simulink model "Inverse_Forward_Simscape"  (R2024b)
settings: Solver=VariableStepAuto  StartTime=0.0  StopTime=10.0  RelTol=1e-3
undefined symbols (not defined in the file or in its folder): smiData, X, Y, Z
libraries: sm_lib x70, nesl_utility x38, robotcorelib x3
(part 2 of 2)

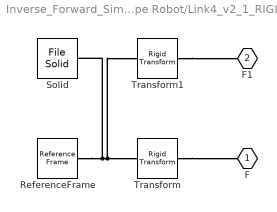
== system Inverse_Forward_Simscape/Simscape Robot/Link4_v2_1_RIGID1 ==
  ReferenceFrame : sm_lib/Frames and Transforms/Reference Frame
  Solid : sm_lib/Body Elements/File Solid  ExtGeomFileName=C:\Users\Chhay\Desktop\simscape\simscape\Solidworks FIle\Link4_v2_Default_sldprt.STEP  UnitType=FromFile  ExtGeomFileUnits=m  StepReaderType=HEX  ExportConvexHullGeometry=off  InertiaType=Custom  BasedOnType=DensityFromFile  Density=1000  DensityUnits=kg/m^3  Mass=smiData.Solid(7).mass  MassUnits=kg  CenterOfMass=smiData.Solid(7).CoM  CenterOfMassUnits=mm  MomentsOfInertia=smiData.Solid(7).MoI  MomentsOfInertiaUnits=kg*mm^2  ProductsOfInertia=smiData.Solid(7).PoI  ProductsOfInertiaUnits=kg*mm^2  GraphicType=FromGeometry  MarkerShape=Sphere  MarkerSize=10  GraphicVisPropType=SimpleVisualProperties  GraphicDiffuseColor=[0.0 1.0 1.0]  GraphicOpacity=smiData.Solid(7).opacity  GraphicSpecularColor=[0.1 0.1 0.1 1.0]  GraphicAmbientColor=[0.15 0.15 0.15 1.0]  GraphicEmissiveColor=[0.5 0.5 0.5 1.0]  GraphicShininess=75  DoExposeReferenceFrame=on  SerializedFrames=<Frames/>
  Transform : sm_lib/Frames and Transforms/Rigid Transform  RotationMethod=ArbitraryAxis  FollAlignAxisA=+X  BaseAlignAxisA=+Y  FollAlignAxisB=+Y  BaseAlignAxisB=+Z  RotationStandardAxis=+Z  RotationAngle=smiData.RigidTransform(2).angle  RotationAngleUnits=rad  RotationArbitraryAxis=smiData.RigidTransform(2).axis  RotationSequenceAxes=FollowerAxes  RotationSequence=XYX  RotationSequenceAngles=[0 0 0]  RotationSequenceAnglesUnits=deg  RotationMatrix=[1 0 0; 0 1 0; 0 0 1]  Quaternion=[1 0 0 0]  TranslationMethod=Cartesian  TranslationCartesianOffset=smiData.RigidTransform(2).translation  TranslationCartesianOffsetUnits=mm  TranslationStandardAxis=+Z  TranslationStandardOffset=0  TranslationStandardOffsetUnits=mm  TranslationROffset=0  TranslationROffsetUnits=m  TranslationThetaOffset=0  TranslationThetaOffsetUnits=deg  TranslationZOffset=0  TranslationZOffsetUnits=m
  Transform1 : sm_lib/Frames and Transforms/Rigid Transform  RotationMethod=ArbitraryAxis  FollAlignAxisA=+X  BaseAlignAxisA=+Y  FollAlignAxisB=+Y  BaseAlignAxisB=+Z  RotationStandardAxis=+Z  RotationAngle=smiData.RigidTransform(3).angle  RotationAngleUnits=rad  RotationArbitraryAxis=smiData.RigidTransform(3).axis  RotationSequenceAxes=FollowerAxes  RotationSequence=XYX  RotationSequenceAngles=[0 0 0]  RotationSequenceAnglesUnits=deg  RotationMatrix=[1 0 0; 0 1 0; 0 0 1]  Quaternion=[1 0 0 0]  TranslationMethod=Cartesian  TranslationCartesianOffset=smiData.RigidTransform(3).translation  TranslationCartesianOffsetUnits=mm  TranslationStandardAxis=+Z  TranslationStandardOffset=0  TranslationStandardOffsetUnits=mm  TranslationROffset=0  TranslationROffsetUnits=m  TranslationThetaOffset=0  TranslationThetaOffsetUnits=deg  TranslationZOffset=0  TranslationZOffsetUnits=m
  F : PMIOPort  Side=Left
  F1 : PMIOPort  Port=2  Side=Right
  connections:
  ReferenceFrame/RConn1 -- Transform/LConn1 -- Transform1/LConn1 -- Solid/RConn1
  Transform/RConn1 -- F/RConn1
  Transform1/RConn1 -- F1/RConn1

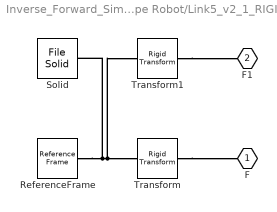
== system Inverse_Forward_Simscape/Simscape Robot/Link5_v2_1_RIGID1 ==
  ReferenceFrame : sm_lib/Frames and Transforms/Reference Frame
  Solid : sm_lib/Body Elements/File Solid  ExtGeomFileName=C:\Users\Chhay\Desktop\simscape\simscape\Solidworks FIle\Link5_v2_Default_sldprt.STEP  UnitType=FromFile  ExtGeomFileUnits=m  StepReaderType=HEX  ExportConvexHullGeometry=off  InertiaType=Custom  BasedOnType=DensityFromFile  Density=1000  DensityUnits=kg/m^3  Mass=smiData.Solid(1).mass  MassUnits=kg  CenterOfMass=smiData.Solid(1).CoM  CenterOfMassUnits=mm  MomentsOfInertia=smiData.Solid(1).MoI  MomentsOfInertiaUnits=kg*mm^2  ProductsOfInertia=smiData.Solid(1).PoI  ProductsOfInertiaUnits=kg*mm^2  GraphicType=FromGeometry  MarkerShape=Sphere  MarkerSize=10  GraphicVisPropType=SimpleVisualProperties  GraphicDiffuseColor=[0.2 1.0 1.0]  GraphicOpacity=smiData.Solid(1).opacity  GraphicSpecularColor=[0.5 0.5 0.5 1.0]  GraphicAmbientColor=[0.15 0.15 0.15 1.0]  GraphicEmissiveColor=[0.0 0.0 0.0 1.0]  GraphicShininess=75  DoExposeReferenceFrame=on  SerializedFrames=<Frames/>
  Transform : sm_lib/Frames and Transforms/Rigid Transform  RotationMethod=ArbitraryAxis  FollAlignAxisA=+X  BaseAlignAxisA=+Y  FollAlignAxisB=+Y  BaseAlignAxisB=+Z  RotationStandardAxis=+Z  RotationAngle=smiData.RigidTransform(4).angle  RotationAngleUnits=rad  RotationArbitraryAxis=smiData.RigidTransform(4).axis  RotationSequenceAxes=FollowerAxes  RotationSequence=XYX  RotationSequenceAngles=[0 0 0]  RotationSequenceAnglesUnits=deg  RotationMatrix=[1 0 0; 0 1 0; 0 0 1]  Quaternion=[1 0 0 0]  TranslationMethod=Cartesian  TranslationCartesianOffset=smiData.RigidTransform(4).translation  TranslationCartesianOffsetUnits=mm  TranslationStandardAxis=+Z  TranslationStandardOffset=0  TranslationStandardOffsetUnits=mm  TranslationROffset=0  TranslationROffsetUnits=m  TranslationThetaOffset=0  TranslationThetaOffsetUnits=deg  TranslationZOffset=0  TranslationZOffsetUnits=m
  Transform1 : sm_lib/Frames and Transforms/Rigid Transform  RotationMethod=ArbitraryAxis  FollAlignAxisA=+X  BaseAlignAxisA=+Y  FollAlignAxisB=+Y  BaseAlignAxisB=+Z  RotationStandardAxis=+Z  RotationAngle=smiData.RigidTransform(9).angle  RotationAngleUnits=rad  RotationArbitraryAxis=smiData.RigidTransform(9).axis  RotationSequenceAxes=FollowerAxes  RotationSequence=XYX  RotationSequenceAngles=[0 0 0]  RotationSequenceAnglesUnits=deg  RotationMatrix=[1 0 0; 0 1 0; 0 0 1]  Quaternion=[1 0 0 0]  TranslationMethod=Cartesian  TranslationCartesianOffset=smiData.RigidTransform(9).translation  TranslationCartesianOffsetUnits=mm  TranslationStandardAxis=+Z  TranslationStandardOffset=0  TranslationStandardOffsetUnits=mm  TranslationROffset=0  TranslationROffsetUnits=m  TranslationThetaOffset=0  TranslationThetaOffsetUnits=deg  TranslationZOffset=0  TranslationZOffsetUnits=m
  F : PMIOPort  Side=Left
  F1 : PMIOPort  Port=2  Side=Right
  connections:
  ReferenceFrame/RConn1 -- Transform/LConn1 -- Transform1/LConn1 -- Solid/RConn1
  Transform/RConn1 -- F/RConn1
  Transform1/RConn1 -- F1/RConn1

== system Inverse_Forward_Simscape/Simscape Robot1/Base_2_RIGID1 ==
  ReferenceFrame : sm_lib/Frames and Transforms/Reference Frame
  Solid : sm_lib/Body Elements/File Solid  ExtGeomFileName=D:\Test_hardware\simscape\Solidworks FIle\Base_Default_sldprt.STEP  UnitType=FromFile  ExtGeomFileUnits=m  StepReaderType=HEX  ExportConvexHullGeometry=off  InertiaType=Custom  Mass=smiData.Solid(5).mass  MassUnits=kg  CenterOfMass=smiData.Solid(5).CoM  CenterOfMassUnits=mm  MomentsOfInertia=smiData.Solid(5).MoI  MomentsOfInertiaUnits=kg*mm^2  ProductsOfInertia=smiData.Solid(5).PoI  ProductsOfInertiaUnits=kg*mm^2  BasedOnType=DensityFromFile  Density=1000  DensityUnits=kg/m^3  DoExposeReferenceFrame=on  SerializedFrames=<Frames/>  GraphicType=FromGeometry  MarkerShape=Sphere  MarkerSize=10  GraphicVisPropType=AdvancedVisualProperties  GraphicDiffuseColor=smiData.Solid(5).color  GraphicSpecularColor=[1.0 1.0 1.0 1.0]  GraphicAmbientColor=[0.4 0.4 0.4 1.0]  GraphicEmissiveColor=[0.1 0.1 0.1 1.0]  GraphicShininess=100  GraphicOpacity=smiData.Solid(5).opacity
  Transform : sm_lib/Frames and Transforms/Rigid Transform  TranslationMethod=Cartesian  TranslationStandardOffset=0  TranslationLengthUnit=mm  TranslationStandardAxis=+Z  TranslationCartesianOffset=smiData.RigidTransform(5).translation  TranslationROffset=0  TranslationROffsetUnits=m  TranslationZOffset=0  TranslationZOffsetUnits=m  TranslationThetaOffset=0  TranslationThetaOffsetUnits=deg  RotationMethod=ArbitraryAxis  RotationAngleUnits=rad  RotationStandardAxis=+Z  RotationAngle=smiData.RigidTransform(5).angle  RotationArbitraryAxis=smiData.RigidTransform(5).axis  FollAlignAxisA=+X  BaseAlignAxisA=+Y  FollAlignAxisB=+Y  BaseAlignAxisB=+Z  RotationSequenceAxes=FollowerAxes  RotationSequence=XYX  RotationSequenceAngles=[0 0 0]  RotationSequenceAnglesUnits=deg  RotationMatrix=[1 0 0; 0 1 0; 0 0 1]  Quaternion=[1 0 0 0]
  F1 : PMIOPort  Side=Left
  F : PMIOPort  Port=2  Side=Right
  connections:
  ReferenceFrame/RConn1 -- Transform/LConn1 -- F1/RConn1 -- Solid/RConn1
  Transform/RConn1 -- F/RConn1

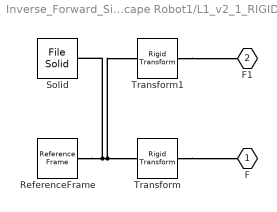
== system Inverse_Forward_Simscape/Simscape Robot1/L1_v2_1_RIGID1 ==
  ReferenceFrame : sm_lib/Frames and Transforms/Reference Frame
  Solid : sm_lib/Body Elements/File Solid  ExtGeomFileName=D:\Test_hardware\simscape\Solidworks FIle\L1_v2_Default_sldprt.STEP  UnitType=FromFile  ExtGeomFileUnits=m  StepReaderType=HEX  ExportConvexHullGeometry=off  InertiaType=Custom  Mass=smiData.Solid(6).mass  MassUnits=kg  CenterOfMass=smiData.Solid(6).CoM  CenterOfMassUnits=mm  MomentsOfInertia=smiData.Solid(6).MoI  MomentsOfInertiaUnits=kg*mm^2  ProductsOfInertia=smiData.Solid(6).PoI  ProductsOfInertiaUnits=kg*mm^2  BasedOnType=DensityFromFile  Density=1000  DensityUnits=kg/m^3  DoExposeReferenceFrame=on  SerializedFrames=<Frames/>  GraphicType=FromGeometry  MarkerShape=Sphere  MarkerSize=10  GraphicVisPropType=SimpleVisualProperties  GraphicDiffuseColor=[0.0 1.0 1.0]  GraphicSpecularColor=[1.0 1.0 1.0 1.0]  GraphicAmbientColor=[0.3 0.30 0.30 1.0]  GraphicEmissiveColor=[0.1 0.1 0.1 1.0]  GraphicShininess=100  GraphicOpacity=smiData.Solid(6).opacity
  Transform : sm_lib/Frames and Transforms/Rigid Transform  TranslationMethod=Cartesian  TranslationStandardOffset=0  TranslationLengthUnit=mm  TranslationStandardAxis=+Z  TranslationCartesianOffset=smiData.RigidTransform(6).translation  TranslationROffset=0  TranslationROffsetUnits=m  TranslationZOffset=0  TranslationZOffsetUnits=m  TranslationThetaOffset=0  TranslationThetaOffsetUnits=deg  RotationMethod=ArbitraryAxis  RotationAngleUnits=rad  RotationStandardAxis=+Z  RotationAngle=smiData.RigidTransform(6).angle  RotationArbitraryAxis=smiData.RigidTransform(6).axis  FollAlignAxisA=+X  BaseAlignAxisA=+Y  FollAlignAxisB=+Y  BaseAlignAxisB=+Z  RotationSequenceAxes=FollowerAxes  RotationSequence=XYX  RotationSequenceAngles=[0 0 0]  RotationSequenceAnglesUnits=deg  RotationMatrix=[1 0 0; 0 1 0; 0 0 1]  Quaternion=[1 0 0 0]
  Transform1 : sm_lib/Frames and Transforms/Rigid Transform  TranslationMethod=Cartesian  TranslationStandardOffset=0  TranslationLengthUnit=mm  TranslationStandardAxis=+Z  TranslationCartesianOffset=smiData.RigidTransform(7).translation  TranslationROffset=0  TranslationROffsetUnits=m  TranslationZOffset=0  TranslationZOffsetUnits=m  TranslationThetaOffset=0  TranslationThetaOffsetUnits=deg  RotationMethod=ArbitraryAxis  RotationAngleUnits=rad  RotationStandardAxis=+Z  RotationAngle=smiData.RigidTransform(7).angle  RotationArbitraryAxis=smiData.RigidTransform(7).axis  FollAlignAxisA=+X  BaseAlignAxisA=+Y  FollAlignAxisB=+Y  BaseAlignAxisB=+Z  RotationSequenceAxes=FollowerAxes  RotationSequence=XYX  RotationSequenceAngles=[0 0 0]  RotationSequenceAnglesUnits=deg  RotationMatrix=[1 0 0; 0 1 0; 0 0 1]  Quaternion=[1 0 0 0]
  F : PMIOPort  Side=Left
  F1 : PMIOPort  Port=2  Side=Right
  connections:
  ReferenceFrame/RConn1 -- Transform/LConn1 -- Transform1/LConn1 -- Solid/RConn1
  Transform/RConn1 -- F/RConn1
  Transform1/RConn1 -- F1/RConn1

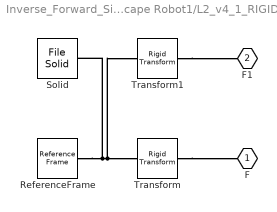
== system Inverse_Forward_Simscape/Simscape Robot1/L2_v4_1_RIGID1 ==
  ReferenceFrame : sm_lib/Frames and Transforms/Reference Frame
  Solid : sm_lib/Body Elements/File Solid  ExtGeomFileName=D:\Test_hardware\simscape\Solidworks FIle\L2_v4_Default_sldprt.STEP  UnitType=FromFile  ExtGeomFileUnits=m  StepReaderType=HEX  ExportConvexHullGeometry=off  InertiaType=Custom  Mass=smiData.Solid(4).mass  MassUnits=kg  CenterOfMass=smiData.Solid(4).CoM  CenterOfMassUnits=mm  MomentsOfInertia=smiData.Solid(4).MoI  MomentsOfInertiaUnits=kg*mm^2  ProductsOfInertia=smiData.Solid(4).PoI  ProductsOfInertiaUnits=kg*mm^2  BasedOnType=DensityFromFile  Density=1000  DensityUnits=kg/m^3  DoExposeReferenceFrame=on  SerializedFrames=<Frames/>  GraphicType=FromGeometry  MarkerShape=Sphere  MarkerSize=10  GraphicVisPropType=SimpleVisualProperties  GraphicDiffuseColor=[0.0 1.0 1.0]  GraphicSpecularColor=[0.5 0.5 0.5 1.0]  GraphicAmbientColor=[0.15 0.15 0.15 1.0]  GraphicEmissiveColor=[0.0 0.0 0.0 1.0]  GraphicShininess=75  GraphicOpacity=smiData.Solid(4).opacity
  Transform : sm_lib/Frames and Transforms/Rigid Transform  TranslationMethod=Cartesian  TranslationStandardOffset=0  TranslationLengthUnit=mm  TranslationStandardAxis=+Z  TranslationCartesianOffset=smiData.RigidTransform(8).translation  TranslationROffset=0  TranslationROffsetUnits=m  TranslationZOffset=0  TranslationZOffsetUnits=m  TranslationThetaOffset=0  TranslationThetaOffsetUnits=deg  RotationMethod=ArbitraryAxis  RotationAngleUnits=rad  RotationStandardAxis=+Z  RotationAngle=smiData.RigidTransform(8).angle  RotationArbitraryAxis=smiData.RigidTransform(8).axis  FollAlignAxisA=+X  BaseAlignAxisA=+Y  FollAlignAxisB=+Y  BaseAlignAxisB=+Z  RotationSequenceAxes=FollowerAxes  RotationSequence=XYX  RotationSequenceAngles=[0 0 0]  RotationSequenceAnglesUnits=deg  RotationMatrix=[1 0 0; 0 1 0; 0 0 1]  Quaternion=[1 0 0 0]
  Transform1 : sm_lib/Frames and Transforms/Rigid Transform  TranslationMethod=Cartesian  TranslationStandardOffset=0  TranslationLengthUnit=mm  TranslationStandardAxis=+Z  TranslationCartesianOffset=smiData.RigidTransform(11).translation  TranslationROffset=0  TranslationROffsetUnits=m  TranslationZOffset=0  TranslationZOffsetUnits=m  TranslationThetaOffset=0  TranslationThetaOffsetUnits=deg  RotationMethod=ArbitraryAxis  RotationAngleUnits=rad  RotationStandardAxis=+Z  RotationAngle=smiData.RigidTransform(11).angle  RotationArbitraryAxis=smiData.RigidTransform(11).axis  FollAlignAxisA=+X  BaseAlignAxisA=+Y  FollAlignAxisB=+Y  BaseAlignAxisB=+Z  RotationSequenceAxes=FollowerAxes  RotationSequence=XYX  RotationSequenceAngles=[0 0 0]  RotationSequenceAnglesUnits=deg  RotationMatrix=[1 0 0; 0 1 0; 0 0 1]  Quaternion=[1 0 0 0]
  F : PMIOPort  Side=Left
  F1 : PMIOPort  Port=2  Side=Right
  connections:
  ReferenceFrame/RConn1 -- Transform/LConn1 -- Transform1/LConn1 -- Solid/RConn1
  Transform/RConn1 -- F/RConn1
  Transform1/RConn1 -- F1/RConn1

== system Inverse_Forward_Simscape/Simscape Robot1/L6_2_RIGID ==
  ReferenceFrame : sm_lib/Frames and Transforms/Reference Frame
  Solid : sm_lib/Body Elements/File Solid  ExtGeomFileName=D:\Test_hardware\simscape\Solidworks FIle\L6_mass_Default_sldprt.STEP  UnitType=FromFile  ExtGeomFileUnits=m  StepReaderType=HEX  ExportConvexHullGeometry=off  InertiaType=Custom  Mass=smiData.Solid(3).mass  MassUnits=kg  CenterOfMass=smiData.Solid(3).CoM  CenterOfMassUnits=mm  MomentsOfInertia=smiData.Solid(3).MoI  MomentsOfInertiaUnits=kg*mm^2  ProductsOfInertia=smiData.Solid(3).PoI  ProductsOfInertiaUnits=kg*mm^2  BasedOnType=DensityFromFile  Density=1000  DensityUnits=kg/m^3  DoExposeReferenceFrame=on  SerializedFrames=<Frames/>  GraphicType=FromGeometry  MarkerShape=Sphere  MarkerSize=10  GraphicVisPropType=AdvancedVisualProperties  GraphicDiffuseColor=[1.0 1.0 1.0]  GraphicSpecularColor=[0.5 0.5 0.5 1.0]  GraphicAmbientColor=[0.4 0.4 0.4 1.0]  GraphicEmissiveColor=[0.0 0.0 0.0 1.0]  GraphicShininess=75  GraphicOpacity=smiData.Solid(3).opacity
  Transform : sm_lib/Frames and Transforms/Rigid Transform  TranslationMethod=Cartesian  TranslationStandardOffset=0  TranslationLengthUnit=mm  TranslationStandardAxis=+Z  TranslationCartesianOffset=smiData.RigidTransform(10).translation  TranslationROffset=0  TranslationROffsetUnits=m  TranslationZOffset=0  TranslationZOffsetUnits=m  TranslationThetaOffset=0  TranslationThetaOffsetUnits=deg  RotationMethod=ArbitraryAxis  RotationAngleUnits=rad  RotationStandardAxis=+Z  RotationAngle=smiData.RigidTransform(10).angle  RotationArbitraryAxis=smiData.RigidTransform(10).axis  FollAlignAxisA=+X  BaseAlignAxisA=+Y  FollAlignAxisB=+Y  BaseAlignAxisB=+Z  RotationSequenceAxes=FollowerAxes  RotationSequence=XYX  RotationSequenceAngles=[0 0 0]  RotationSequenceAnglesUnits=deg  RotationMatrix=[1 0 0; 0 1 0; 0 0 1]  Quaternion=[1 0 0 0]
  F : PMIOPort  Side=Left
  connections:
  ReferenceFrame/RConn1 -- Solid/RConn1 -- Transform/LConn1
  Transform/RConn1 -- F/RConn1

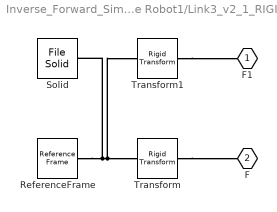
== system Inverse_Forward_Simscape/Simscape Robot1/Link3_v2_1_RIGID1 ==
  ReferenceFrame : sm_lib/Frames and Transforms/Reference Frame
  Solid : sm_lib/Body Elements/File Solid  ExtGeomFileName=D:\Test_hardware\simscape\Solidworks FIle\Link3_v2_Default_sldprt.STEP  UnitType=FromFile  ExtGeomFileUnits=m  StepReaderType=HEX  ExportConvexHullGeometry=off  InertiaType=Custom  Mass=smiData.Solid(2).mass  MassUnits=kg  CenterOfMass=smiData.Solid(2).CoM  CenterOfMassUnits=mm  MomentsOfInertia=smiData.Solid(2).MoI  MomentsOfInertiaUnits=kg*mm^2  ProductsOfInertia=smiData.Solid(2).PoI  ProductsOfInertiaUnits=kg*mm^2  BasedOnType=DensityFromFile  Density=1000  DensityUnits=kg/m^3  DoExposeReferenceFrame=on  SerializedFrames=<Frames/>  GraphicType=FromGeometry  MarkerShape=Sphere  MarkerSize=10  GraphicVisPropType=SimpleVisualProperties  GraphicDiffuseColor=[0.2 1.0 1.0]  GraphicSpecularColor=[0.5 0.5 0.5 1.0]  GraphicAmbientColor=[0.15 0.15 0.15 1.0]  GraphicEmissiveColor=[0.0 0.0 0.0 1.0]  GraphicShininess=75  GraphicOpacity=smiData.Solid(2).opacity
  Transform : sm_lib/Frames and Transforms/Rigid Transform  TranslationMethod=Cartesian  TranslationStandardOffset=0  TranslationLengthUnit=mm  TranslationStandardAxis=+Z  TranslationCartesianOffset=smiData.RigidTransform(1).translation  TranslationROffset=0  TranslationROffsetUnits=m  TranslationZOffset=0  TranslationZOffsetUnits=m  TranslationThetaOffset=0  TranslationThetaOffsetUnits=deg  RotationMethod=ArbitraryAxis  RotationAngleUnits=rad  RotationStandardAxis=+Z  RotationAngle=smiData.RigidTransform(1).angle  RotationArbitraryAxis=smiData.RigidTransform(1).axis  FollAlignAxisA=+X  BaseAlignAxisA=+Y  FollAlignAxisB=+Y  BaseAlignAxisB=+Z  RotationSequenceAxes=FollowerAxes  RotationSequence=XYX  RotationSequenceAngles=[0 0 0]  RotationSequenceAnglesUnits=deg  RotationMatrix=[1 0 0; 0 1 0; 0 0 1]  Quaternion=[1 0 0 0]
  Transform1 : sm_lib/Frames and Transforms/Rigid Transform  TranslationMethod=Cartesian  TranslationStandardOffset=0  TranslationLengthUnit=mm  TranslationStandardAxis=+Z  TranslationCartesianOffset=smiData.RigidTransform(12).translation  TranslationROffset=0  TranslationROffsetUnits=m  TranslationZOffset=0  TranslationZOffsetUnits=m  TranslationThetaOffset=0  TranslationThetaOffsetUnits=deg  RotationMethod=ArbitraryAxis  RotationAngleUnits=rad  RotationStandardAxis=+Z  RotationAngle=smiData.RigidTransform(12).angle  RotationArbitraryAxis=smiData.RigidTransform(12).axis  FollAlignAxisA=+X  BaseAlignAxisA=+Y  FollAlignAxisB=+Y  BaseAlignAxisB=+Z  RotationSequenceAxes=FollowerAxes  RotationSequence=XYX  RotationSequenceAngles=[0 0 0]  RotationSequenceAnglesUnits=deg  RotationMatrix=[1 0 0; 0 1 0; 0 0 1]  Quaternion=[1 0 0 0]
  F1 : PMIOPort  Side=Left
  F : PMIOPort  Port=2  Side=Right
  connections:
  ReferenceFrame/RConn1 -- Transform/LConn1 -- Transform1/LConn1 -- Solid/RConn1
  Transform/RConn1 -- F/RConn1
  Transform1/RConn1 -- F1/RConn1

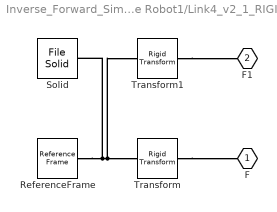
== system Inverse_Forward_Simscape/Simscape Robot1/Link4_v2_1_RIGID1 ==
  ReferenceFrame : sm_lib/Frames and Transforms/Reference Frame
  Solid : sm_lib/Body Elements/File Solid  ExtGeomFileName=D:\Test_hardware\simscape\Solidworks FIle\Link4_v2_Default_sldprt.STEP  UnitType=FromFile  ExtGeomFileUnits=m  StepReaderType=HEX  ExportConvexHullGeometry=off  InertiaType=Custom  Mass=smiData.Solid(7).mass  MassUnits=kg  CenterOfMass=smiData.Solid(7).CoM  CenterOfMassUnits=mm  MomentsOfInertia=smiData.Solid(7).MoI  MomentsOfInertiaUnits=kg*mm^2  ProductsOfInertia=smiData.Solid(7).PoI  ProductsOfInertiaUnits=kg*mm^2  BasedOnType=DensityFromFile  Density=1000  DensityUnits=kg/m^3  DoExposeReferenceFrame=on  SerializedFrames=<Frames/>  GraphicType=FromGeometry  MarkerShape=Sphere  MarkerSize=10  GraphicVisPropType=SimpleVisualProperties  GraphicDiffuseColor=[0.0 1.0 1.0]  GraphicSpecularColor=[0.1 0.1 0.1 1.0]  GraphicAmbientColor=[0.15 0.15 0.15 1.0]  GraphicEmissiveColor=[0.5 0.5 0.5 1.0]  GraphicShininess=75  GraphicOpacity=smiData.Solid(7).opacity
  Transform : sm_lib/Frames and Transforms/Rigid Transform  TranslationMethod=Cartesian  TranslationStandardOffset=0  TranslationLengthUnit=mm  TranslationStandardAxis=+Z  TranslationCartesianOffset=smiData.RigidTransform(2).translation  TranslationROffset=0  TranslationROffsetUnits=m  TranslationZOffset=0  TranslationZOffsetUnits=m  TranslationThetaOffset=0  TranslationThetaOffsetUnits=deg  RotationMethod=ArbitraryAxis  RotationAngleUnits=rad  RotationStandardAxis=+Z  RotationAngle=smiData.RigidTransform(2).angle  RotationArbitraryAxis=smiData.RigidTransform(2).axis  FollAlignAxisA=+X  BaseAlignAxisA=+Y  FollAlignAxisB=+Y  BaseAlignAxisB=+Z  RotationSequenceAxes=FollowerAxes  RotationSequence=XYX  RotationSequenceAngles=[0 0 0]  RotationSequenceAnglesUnits=deg  RotationMatrix=[1 0 0; 0 1 0; 0 0 1]  Quaternion=[1 0 0 0]
  Transform1 : sm_lib/Frames and Transforms/Rigid Transform  TranslationMethod=Cartesian  TranslationStandardOffset=0  TranslationLengthUnit=mm  TranslationStandardAxis=+Z  TranslationCartesianOffset=smiData.RigidTransform(3).translation  TranslationROffset=0  TranslationROffsetUnits=m  TranslationZOffset=0  TranslationZOffsetUnits=m  TranslationThetaOffset=0  TranslationThetaOffsetUnits=deg  RotationMethod=ArbitraryAxis  RotationAngleUnits=rad  RotationStandardAxis=+Z  RotationAngle=smiData.RigidTransform(3).angle  RotationArbitraryAxis=smiData.RigidTransform(3).axis  FollAlignAxisA=+X  BaseAlignAxisA=+Y  FollAlignAxisB=+Y  BaseAlignAxisB=+Z  RotationSequenceAxes=FollowerAxes  RotationSequence=XYX  RotationSequenceAngles=[0 0 0]  RotationSequenceAnglesUnits=deg  RotationMatrix=[1 0 0; 0 1 0; 0 0 1]  Quaternion=[1 0 0 0]
  F : PMIOPort  Side=Left
  F1 : PMIOPort  Port=2  Side=Right
  connections:
  ReferenceFrame/RConn1 -- Transform/LConn1 -- Transform1/LConn1 -- Solid/RConn1
  Transform/RConn1 -- F/RConn1
  Transform1/RConn1 -- F1/RConn1

== system Inverse_Forward_Simscape/Simscape Robot1/Link5_v2_1_RIGID1 ==
  ReferenceFrame : sm_lib/Frames and Transforms/Reference Frame
  Solid : sm_lib/Body Elements/File Solid  ExtGeomFileName=D:\Test_hardware\simscape\Solidworks FIle\Link5_v2_Default_sldprt.STEP  UnitType=FromFile  ExtGeomFileUnits=m  StepReaderType=HEX  ExportConvexHullGeometry=off  InertiaType=Custom  Mass=smiData.Solid(1).mass  MassUnits=kg  CenterOfMass=smiData.Solid(1).CoM  CenterOfMassUnits=mm  MomentsOfInertia=smiData.Solid(1).MoI  MomentsOfInertiaUnits=kg*mm^2  ProductsOfInertia=smiData.Solid(1).PoI  ProductsOfInertiaUnits=kg*mm^2  BasedOnType=DensityFromFile  Density=1000  DensityUnits=kg/m^3  DoExposeReferenceFrame=on  SerializedFrames=<Frames/>  GraphicType=FromGeometry  MarkerShape=Sphere  MarkerSize=10  GraphicVisPropType=SimpleVisualProperties  GraphicDiffuseColor=[0.2 1.0 1.0]  GraphicSpecularColor=[0.5 0.5 0.5 1.0]  GraphicAmbientColor=[0.15 0.15 0.15 1.0]  GraphicEmissiveColor=[0.0 0.0 0.0 1.0]  GraphicShininess=75  GraphicOpacity=smiData.Solid(1).opacity
  Transform : sm_lib/Frames and Transforms/Rigid Transform  TranslationMethod=Cartesian  TranslationStandardOffset=0  TranslationLengthUnit=mm  TranslationStandardAxis=+Z  TranslationCartesianOffset=smiData.RigidTransform(4).translation  TranslationROffset=0  TranslationROffsetUnits=m  TranslationZOffset=0  TranslationZOffsetUnits=m  TranslationThetaOffset=0  TranslationThetaOffsetUnits=deg  RotationMethod=ArbitraryAxis  RotationAngleUnits=rad  RotationStandardAxis=+Z  RotationAngle=smiData.RigidTransform(4).angle  RotationArbitraryAxis=smiData.RigidTransform(4).axis  FollAlignAxisA=+X  BaseAlignAxisA=+Y  FollAlignAxisB=+Y  BaseAlignAxisB=+Z  RotationSequenceAxes=FollowerAxes  RotationSequence=XYX  RotationSequenceAngles=[0 0 0]  RotationSequenceAnglesUnits=deg  RotationMatrix=[1 0 0; 0 1 0; 0 0 1]  Quaternion=[1 0 0 0]
  Transform1 : sm_lib/Frames and Transforms/Rigid Transform  TranslationMethod=Cartesian  TranslationStandardOffset=0  TranslationLengthUnit=mm  TranslationStandardAxis=+Z  TranslationCartesianOffset=smiData.RigidTransform(9).translation  TranslationROffset=0  TranslationROffsetUnits=m  TranslationZOffset=0  TranslationZOffsetUnits=m  TranslationThetaOffset=0  TranslationThetaOffsetUnits=deg  RotationMethod=ArbitraryAxis  RotationAngleUnits=rad  RotationStandardAxis=+Z  RotationAngle=smiData.RigidTransform(9).angle  RotationArbitraryAxis=smiData.RigidTransform(9).axis  FollAlignAxisA=+X  BaseAlignAxisA=+Y  FollAlignAxisB=+Y  BaseAlignAxisB=+Z  RotationSequenceAxes=FollowerAxes  RotationSequence=XYX  RotationSequenceAngles=[0 0 0]  RotationSequenceAnglesUnits=deg  RotationMatrix=[1 0 0; 0 1 0; 0 0 1]  Quaternion=[1 0 0 0]
  F : PMIOPort  Side=Left
  F1 : PMIOPort  Port=2  Side=Right
  connections:
  ReferenceFrame/RConn1 -- Transform/LConn1 -- Transform1/LConn1 -- Solid/RConn1
  Transform/RConn1 -- F/RConn1
  Transform1/RConn1 -- F1/RConn1

== matlab function Inverse_Forward_Simscape/Inverse Kinematics ==
  data: Px input; theta1 output double size=[1,1]; Py input; Pz input; theta2 output double size=[1,1]; theta3 output double size=[1,1]; theta4 output double size=[1,1]; theta5 output double size=[1,1]; theta6 output double size=[1,1]; initialGuess_1 input
function [theta1, theta2, theta3, theta4, theta5, theta6] = fcn(Px, Py, Pz, initialGuess_1)
    % Enter orientation of our end effector
    % This is an examplar orientation which is always pointing to the
    % right%
    R0_6 = [0 0 1
            0 -1 0
            1 0 0];
  
    % Find the position of the wrist
    % From end effector to the wrist, the distance is 108mm
    d6 = 108;

    % r13 is the cos of angle between the x axis of end effector
    % and z axis of base
    r13 = R0_6(1,3);

    % r23 is the cos of angle between the y axis of end effector
    % and z axis of base
    r23 = R0_6(2,3);

    % r33 is the cos of angle between the z axis of end effector
    % and z axis of base
    r33 = R0_6(3,3);

    Wx = Px - d6 * r13;
    Wy = Py - d6 * r23;
    Wz = Pz - d6 * r33;

    r = sqrt((Wx)^2 + (Wy)^2);
    s = Wz - 276;

    % Find theta1 using the position of the wrist
    % Using projection onto x and y plane
    theta1 = -(atan(Wy / Wx));

    % Define the system of equations for theta2 and theta3
    function F = equations(vars)
        theta2 = vars(1);
        theta3 = vars(2);
        F = zeros(2, 1);  % Ensure F is defined correctly as a column vector
        
        % Equations
        F(1) = r - (306*sin(theta2) + 79.75*sin(theta2+theta3) + 387*cos(theta2+theta3));
        F(2) = s - (306*cos(theta2) + 79.75*cos(theta2+theta3) - 387*sin(theta2+theta3));


    end

    % Initial guesses for theta2 and theta3
    initialGuess = [0.1, 0];

    % Use fsolve with the 'levenberg-marquardt' algorithm
    options = optimoptions('fsolve', 'Algorithm', 'levenberg-marquardt', 'Display', 'none');
    vars = fsolve(@equations, initialGuess, options);

    % Assign output variables
    
  if vars(1)>pi/2
      theta2 = pi/2;
  elseif vars(1)<-pi/2
      theta2 = -pi/2;
  else
      theta2 = vars(1);
  end

  if vars(2)>1.1
      theta3 = -1.1;
  elseif vars(2)<-1.1
      theta3 = 1.1;
  else 
      theta3 = -vars(2);
  end

    %From forward kinematics 
    %refer to file rotationmatrix.mlx
    %Find the appropriate equations then paste them in the equations list
    %below

    function G = equa(thet)
        theta4 = thet(1);
        theta5 = thet(2);
        theta6 = thet(3);
        G = zeros(5, 1);  % Ensure F is defined correctly as a column vector
        
        % Equations
if theta1 == 0
        G(3) = cos(theta1)*sin(theta2)*sin(theta3) - cos(theta5) + cos(theta1)*cos(theta2)*cos(theta3);      
        G(4) = - sin(theta5)*sin(theta6) - sin(theta1)*sin(theta2)*sin(theta3) - cos(theta2)*cos(theta3)*sin(theta1);      
        G(5) = cos(theta2)*sin(theta3) - cos(theta3)*sin(theta2) - cos(theta6)*sin(theta5);
        

elseif theta1 ~= 0 && theta1 < 1.309 && theta1 > -1.309
        G(1) =  - sin(theta1) - sin(theta4)*sin(theta5);
        G(2) =  cos(theta4)*cos(theta6) - cos(theta1) + cos(theta5)*sin(theta4)*sin(theta6);
        G(3) =  cos(theta5)*cos(theta6)*sin(theta4) - cos(theta4)*sin(theta6);
        G(4) = cos(theta1)*sin(theta2)*sin(theta3) - cos(theta5) + cos(theta1)*cos(theta2)*cos(theta3);
        G(5) = cos(theta2)*sin(theta3) - cos(theta3)*sin(theta2) - cos(theta6)*sin(theta5);

end
end

    % Use fsolve with the 'levenberg-marquardt' algorithm
    options_1 = optimoptions('fsolve', 'Algorithm', 'levenberg-marquardt', 'Display', 'none');
    thet = fsolve(@equa, initialGuess_1, options_1);


    % Assign output variables
    theta4 = thet(1);
    theta5 = thet(2);
    theta6 = thet(3);
    
    
 
 


    

end

== matlab function Inverse_Forward_Simscape/Forward Kinematics ==
  data: Px output; t1 input double size=[1,1]; t2 input double size=[1,1]; t3 input double size=[1,1]; t4 input double size=[1,1]; t5 input double size=[1,1]; t6 input double size=[1,1]; Py output; Pz output; Tr output
function [Px,Py,Pz,Tr] = fcn(t1,t2,t3,t4,t5,t6)


theta1 = t1;        d1 = 276;   a1 = 0;         alpha1 = -pi/2;
theta2 = t2-pi/2;   d2 = 0;     a2 = 306;       alpha2 = 0;
theta3 = t3;        d3 = 0;     a3 = 79.75;     alpha3 = -pi/2;
theta4 = 0;         d4 = 160;   a4 = 0;         alpha4 = 0;         %fixed Frame%
theta5 = t4;        d5 = 227;   a5 = 0;         alpha5 = pi/2;
theta6 = t5;        d6 = 0;     a6 = 0;         alpha6 = -pi/2;
theta7 = 0;         d7 = 70;    a7 = 0;         alpha7 = 0;         %Fixed Frame%
theta8 = t6;        d8 = 38;    a8 = 0;         alpha8 = 0;


%from 1 to 2%
T_1 = [cos(theta1), -cos(alpha1)*sin(theta1),  sin(alpha1)*sin(theta1), a1*cos(theta1)
       sin(theta1),  cos(alpha1)*cos(theta1), -sin(alpha1)*cos(theta1), a1*sin(theta1)
                0,             sin(alpha1),             cos(alpha1),            d1
                0,                      0,                      0,            1];

%from 2 to 3%
T_2 = [cos(theta2), -cos(alpha2)*sin(theta2),  sin(alpha2)*sin(theta2), a2*cos(theta2)
      sin(theta2),  cos(alpha2)*cos(theta2), -sin(alpha2)*cos(theta2), a2*sin(theta2)
               0,             sin(alpha2),             cos(alpha2),            d2
               0,                      0,                      0,            1];

%from 3 to 4%
T_3 = [cos(theta3), -cos(alpha3)*sin(theta3),  sin(alpha3)*sin(theta3), a3*cos(theta3)
      sin(theta3),  cos(alpha3)*cos(theta3), -sin(alpha3)*cos(theta3), a3*sin(theta3)
               0,             sin(alpha3),             cos(alpha3),            d3
               0,                      0,                      0,            1];

%from 4 to 5%
T_4 = [cos(theta4), -cos(alpha1)*sin(theta4),  sin(alpha4)*sin(theta4), a4*cos(theta4)
      sin(theta4),  cos(alpha1)*cos(theta4), -sin(alpha4)*cos(theta4), a4*sin(theta4)
               0,             sin(alpha4),             cos(alpha4),            d4
               0,                      0,                      0,            1];

%from 5 to 6%
T_5 = [cos(theta5), -cos(alpha5)*sin(theta5),  sin(alpha5)*sin(theta5), a5*cos(theta5)
      sin(theta5),  cos(alpha5)*cos(theta5), -sin(alpha5)*cos(theta5), a5*sin(theta5)
               0,             sin(alpha5),             cos(alpha5),            d5
               0,                      0,                      0,            1];

%from 6 to 7%
T_6 = [cos(theta6), -cos(alpha6)*sin(theta6),  sin(alpha6)*sin(theta6), a6*cos(theta6)
      sin(theta6),  cos(alpha6)*cos(theta6), -sin(alpha6)*cos(theta6), a6*sin(theta6)
               0,             sin(alpha6),             cos(alpha6),            d6
               0,                      0,                      0,            1];

%from 7 to 8%
T_7 = [cos(theta7), -cos(alpha7)*sin(theta7),  sin(alpha7)*sin(theta7), a7*cos(theta7)
      sin(theta7),  cos(alpha7)*cos(theta7), -sin(alpha7)*cos(theta7), a7*sin(theta7)
               0,             sin(alpha7),             cos(alpha7),            d7
               0,                      0,                      0,            1];

%from 8 to 9%
T_8 = [cos(theta8), -cos(alpha8)*sin(theta8),  sin(alpha8)*sin(theta8), a8*cos(theta8)
      sin(theta8),  cos(alpha8)*cos(theta8), -sin(alpha8)*cos(theta8), a8*sin(theta8)
               0,             sin(alpha8),             cos(alpha8),            d8
               0,                      0,                      0,            1];


Tr = T_1*T_2*T_3*T_4*T_5*T_6*T_7*T_8;
Px = Tr(1,4);
Py = Tr(2,4);
Pz = Tr(3,4);
end

== matlab function Inverse_Forward_Simscape/Forward_Kinematic_Good1 ==
  data: Px output; Py output; Pz output; th1 input; th2 input; th3 input; th4 input; th5 input; th6 input
function [Px,Py,Pz] = forward_kinematics(th1, th2, th3, th4, th5, th6)
%All length in mm
l1=276;
l2=306;
a=79.75;
l3=160;
l4=227;
l5=70;
l6=38;
    % Compute DH transformation matrices
    A0 = dh_matrix(0    , 0     ,l1 , th1);   
    A1 = dh_matrix(0    ,-pi/2  ,0  , th2-pi/2);
    A2 = dh_matrix(l2   ,0      ,0  ,th3);
%     A3p= dh_matrix(a   ,0      ,0, 0);
    A3 = dh_matrix(a    ,-pi/2  ,0  ,th4);
    A4 = dh_matrix(0    ,0      ,l3+l4 ,0);
    A4p= dh_matrix(0   ,pi/2   ,0  ,th5);
    A5 = dh_matrix(0    ,-pi/2  , 0 ,th6);
    A6 = dh_matrix(0    ,0      ,l5+l6 ,0);
    
    % Total forward matrix H
    A0_6 = ( A0*A1 * A2 * A3 * A4 * A4p * A5 * A6) ;
    Px=A0_6(1,4);
    Py=A0_6(2,4);
    Pz=A0_6(3,4);

end
function A = dh_matrix(a , alpha ,d ,theta)
    A = [cos(theta)            , -sin(theta),           0       ,   a;
         cos(alpha)*sin(theta), cos(theta)*cos(alpha), -sin(alpha), -d*sin(alpha);
         sin(alpha)*sin(theta), sin(alpha)*cos(theta), cos(alpha), d*cos(alpha);
         0, 0, 0, 1];
end

== matlab function Inverse_Forward_Simscape/Inverse Kinematic ==
  settings: updateMethod=DISCRETE
  data: Px input; q1 output; Py input; Pz input; q2 output; q3 output; q4 output; q5 output; q6 output; R06 input
function [q1, q2, q3, q4, q5, q6] = inverseKinematics(Px, Py, Pz, R06)
    % Define actual geometry parameters (in mm)
%     l1=276;
%     l2=306;
%     a=79.75;
%     l3=160;
%     l4=227;
%     l5=70;
%     l6=38;
    % Wrist position calculation
    O6=[Px,Py,Pz]';
    d6=l5+l6;
    OW = O6 - R06*[0;0;d6];
    % Compute wrist position (compensating for the end-effector offset)
    Pwx=OW(1);
    Pwy=OW(2);
    Pwz=OW(3);
    % Compute q1 directly from the wrist position
    q1 = atan2(Pwy, Pwx);
    r = sqrt(Pwx^2 + Pwy^2);
    h= Pwz-l1;
    % Intermediate calculations for q2 and q3
    s = sqrt(h^2 + r^2);
    alp = atan(h/r );
    w3 = l3 + l4;
    k3 = sqrt(a^2 + w3^2);
    beta = acos((l2^2 + s^2 - k3^2) / (2 * l2 * s));
    gamma = acos(( l2^2+k3^2-s^2) / (2 * l2 * k3));
    Phi = atan(w3/a);
    % Target angles for q2 and q3
    q2 = (-alp -beta+pi/2);
    q3 = (pi-gamma - Phi);

    % Compute R0_3 from q1, q2, q3
    R03 = [cos(q1)*cos(q2 + q3), -cos(q1)*sin(q2 + q3), -sin(q1);
           sin(q1)*cos(q2 + q3), -sin(q1)*sin(q2 + q3),  cos(q1);
           -sin(q2 + q3)       , -cos(q2 + q3)        , 0 ];
    R03t=transpose(R03);

    % Compute R3_6 from the known R0_3 and R0_6
    R3_6 = R03t* R06;

    % Extract elements from R3_6 for calculating q4, q5, q6
    s5c4 = -R3_6(1, 3);
    c5   = R3_6(2, 3);
    s5s4 = R3_6(3, 3);
    s5c6 = R3_6(2, 1);
    s5s6 = -R3_6(2, 2);

    % Joint angle q5

      q5p = atan2(-sqrt(1-c5^2),c5);
 % Joint angles q4 and q6
      q5=q5p;
        q4 = atan2(-s5s4, -s5c4);
        q6 = atan2(-s5s6, -s5c6);

end
